simulink model "nablyudayuschee_ustroistvo"  (Simulink 7.7)
settings: Solver=ode45  StartTime=0.0  StopTime=10.0  RelTol=1e-3
values from neighbouring files (symbols this model uses):
  A = [0 0; 1 0]    [observer_Fi.m]    (also in observer_Psi.m; observer_Z.m)
  C = [0 1]    [observer_Fi.m]    (also in observer_Psi.m; observer_Z.m)
  K = place(A,B,[p1 p2])    [observer_Fi.m]    (also in observer_Psi.m; observer_Z.m)
undefined symbols (not defined in the file or in its folder): KC
settings Model: Creator=Alexey  LastModifiedBy=Alexey

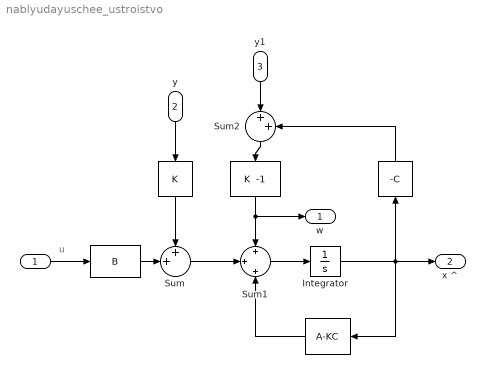
== system nablyudayuschee_ustroistvo ==
  note: u
  "  " : Inport
  y : Inport  Port=2
  y1 : Inport  Port=3
  " " : Fcn  Expr=B
  "    " : Fcn  Expr=K
  "        " : Fcn  Expr=A-KC
  "         " : Fcn  Expr=-C
  "           " : Fcn  Expr="K  -1"
  Integrator : Integrator
  Sum : Sum  Inputs=++|
  Sum1 : Sum  Inputs=+|+|+
  Sum2 : Sum  Inputs=|++
  w : Outport
  x ^ : Outport  Port=2
  wires:
  "  "/1 -> " "/1
  " "/1 -> Sum/2
  Sum/1 -> Sum1/2
  Sum1/1 -> Integrator/1
  Integrator/1 -> "         "/1, "        "/1, x ^/1
  "    "/1 -> Sum/1
  y/1 -> "    "/1
  "           "/1 -> Sum1/1, w/1
  Sum2/1 -> "           "/1
  y1/1 -> Sum2/1
  "         "/1 -> Sum2/2
  "        "/1 -> Sum1/3
